simulink model "Kubon_lab8_2_sim"  (R2020b)
settings: Solver=VariableStepAuto  StartTime=0.0  StopTime=100.0  RelTol=1e-3
values from neighbouring files (symbols this model uses):
  d1 = 0.1*fwe1max    [Kubon_lab6.m]    (also in Kubon_lab7.m = 0; Kubon_lab8.m = 0)
  d2 = 0.1*fwe2max    [Kubon_lab6.m]    (also in Kubon_lab7.m; Kubon_lab8.m)
  h10 = fwe1/a1    [Kubon_lab6.m]    (also in Kubon_lab6_test.m; Kubon_lab7.m = (1/(2*g))*(fwe1/Aw1)^2 + (1/(2*g))*(((fwe2+fwe1)/Aw2)^2); Kubon_lab8.m = fwe1/a1+(fwe2+fwe1)/a2)
  h20 = (fwe1+fwe2)/a2    [Kubon_lab6.m]    (also in Kubon_lab6_test.m; Kubon_lab7.m = 1/(2*g)*(((fwe1+fwe2)/Aw2)^2); Kubon_lab8.m = (fwe2+fwe1)/a2)
  L1 = [(Cv2*a_1) (a_1*(ks2+a_1+k0))]    [Kubon_lab10.m]    (also in Kubon_lab8.m = M2_)
  L2 = [(Cv2*ks1) ((k0*ks2)+(ks1*(a_1+ks2+k0)))]    [Kubon_lab10.m]    (also in Kubon_lab8.m = [ a1 ])
  L3 = (k0*a_1+a_1*a_1)    (= 1108800)    [Kubon_lab10.m]    (also in Kubon_lab8.m = [ a1 ])
  L4 = [(Cv1+ks2) (k0*ks1+(a_1*ks1)+(ks2*(a_1+ks1+k0)))]    [Kubon_lab10.m]    (also in Kubon_lab8.m = M1_)
  M1 = [(Cv1*Cv2) (Cv1*a_1+Cv1*ks2+Cv1*k0+Cv2*a_1+Cv2*ks1+Cv2*k0) (a_1^2+a_1*ks2+a_1*k0  +a_1*ks1+ks1*ks2+ks1*k0    +k0*ks2)]    [Kubon_lab10.m]    (also in Kubon_lab8.m = [A1*A2 , A1*a1+A1*a2+A2*a1 , a1*a2])
  M2 = M1    [Kubon_lab10.m]    (also in Kubon_lab8.m)
  M3 = M2    [Kubon_lab10.m]    (also in Kubon_lab8.m)
  M4 = M3    [Kubon_lab10.m]    (also in Kubon_lab8.m)
  t0 = 50.0    (= 50)    [Kubon_lab10.m]    (also in Kubon_lab4.m = 5; Kubon_lab5.m = 0; Kubon_lab6.m = 5; Kubon_lab6_test.m = 0)
settings Model: Creator=pkubo  LastModifiedBy=pkubo

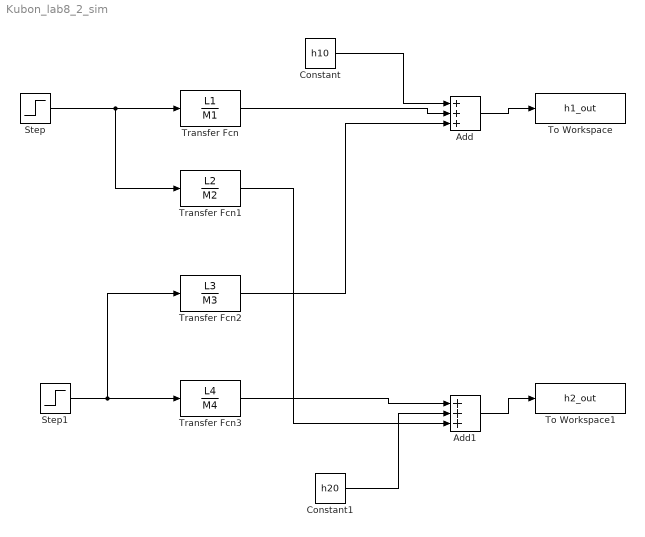
== system Kubon_lab8_2_sim ==
  Add : Sum  Inputs=+++
  Add1 : Sum  Inputs=+++
  Constant : Constant  Value=h10
  Constant1 : Constant  Value=h20
  Step : Step  Time=t0  After=d1  SampleTime=0
  Step1 : Step  Time=t0  After=d2  SampleTime=0
  To Workspace : ToWorkspace  VariableName=h1_out  SampleTime=-1
  To Workspace1 : ToWorkspace  VariableName=h2_out  SampleTime=-1
  Transfer Fcn : TransferFcn  Numerator=L1  Denominator=M1
  Transfer Fcn1 : TransferFcn  Numerator=L2  Denominator=M2
  Transfer Fcn2 : TransferFcn  Numerator=L3  Denominator=M3
  Transfer Fcn3 : TransferFcn  Numerator=L4  Denominator=M4
  wires:
  Add/1 -> To Workspace/1
  Add1/1 -> To Workspace1/1
  Transfer Fcn/1 -> Add/2
  Constant/1 -> Add/1
  Step/1 -> Transfer Fcn1/1, Transfer Fcn/1
  Step1/1 -> Transfer Fcn2/1, Transfer Fcn3/1
  Constant1/1 -> Add1/2
  Transfer Fcn3/1 -> Add1/1
  Transfer Fcn2/1 -> Add/3
  Transfer Fcn1/1 -> Add1/3
